simulink model "Timer"  (R2019b)
settings: Solver=VariableStepAuto  StartTime=0.0  StopTime=10.0  RelTol=1e-3
libraries: powerlib_meascontrol x1
settings Model: Creator=YJR  LastModifiedBy=YJR

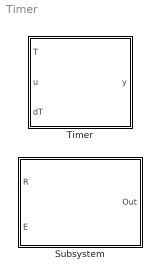
== system Timer ==
  Subsystem : Subsystem  mask(CounterEnabled){}
      mask help: Count the number of square waves.
      mask Display: disp('CounterEnabled')
  Timer : Subsystem  mask(Time Count){}
      mask help: The timer starts when it is triggered, and it is output after a set time. You can set the duration and time step.
      mask Display: disp('Timer')

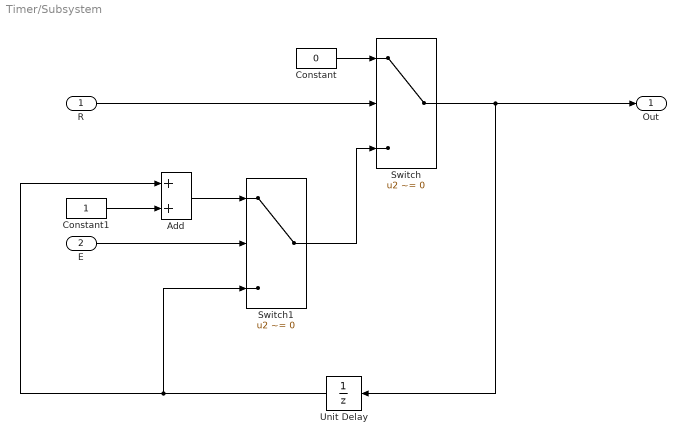
== system Timer/Subsystem ==
  R : Inport
  E : Inport  Port=2
  Add : Sum
  Constant : Constant  Value=0
  Constant1 : Constant
  Switch : Switch  Criteria=u2 ~= 0
  Switch1 : Switch  Criteria=u2 ~= 0
  Unit Delay : UnitDelay  SampleTime=-1  HasFrameUpgradeWarning=on
  Out : Outport
  wires:
  Constant/1 -> Switch/1
  Switch1/1 -> Switch/3
  Switch/1 -> Out/1, Unit Delay/1
  Add/1 -> Switch1/1
  R/1 -> Switch/2
  E/1 -> Switch1/2
  Unit Delay/1 -> Switch1/3, Add/1
  Constant1/1 -> Add/2

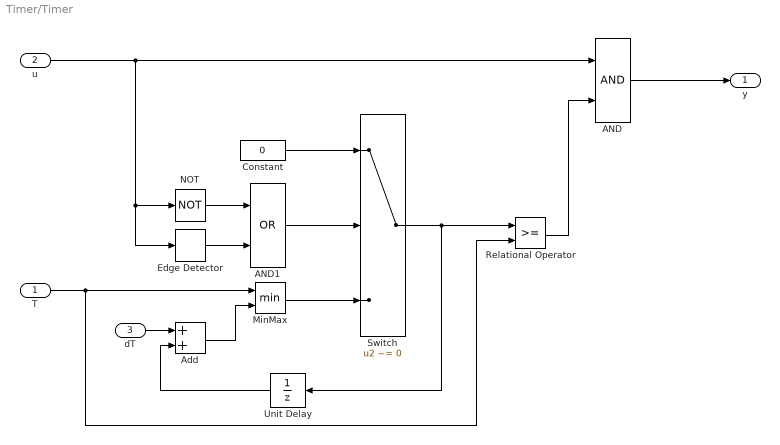
== system Timer/Timer ==
  T : Inport
  u : Inport  Port=2
  dT : Inport  Port=3
  AND : Logic  AllPortsSameDT=off  OutDataTypeStr=boolean
  AND1 : Logic  Operator=OR  AllPortsSameDT=off  OutDataTypeStr=boolean
  Add : Sum
  Constant : Constant  Value=0
  Edge Detector : powerlib_meascontrol/Logic/Edge Detector  model=Rising  ic=0  Ts=-1
      settings: SourceProductName=Simscape Electrical  SourceProductBaseCode=PS
  MinMax : MinMax  Inputs=2
  NOT : Logic  Operator=NOT  AllPortsSameDT=off  OutDataTypeStr=boolean
  Relational Operator : RelationalOperator  OutDataTypeStr=boolean  RndMeth=Simplest
  Switch : Switch  Criteria=u2 ~= 0
  Unit Delay : UnitDelay  SampleTime=-1  HasFrameUpgradeWarning=on
  y : Outport
  wires:
  Edge Detector/1 -> AND1/2
  u/1 -> Edge Detector/1, NOT/1, AND/1
  AND/1 -> y/1
  Unit Delay/1 -> Add/2
  Add/1 -> MinMax/2
  dT/1 -> Add/1
  Switch/1 -> Relational Operator/1, Unit Delay/1
  NOT/1 -> AND1/1
  T/1 -> MinMax/1, Relational Operator/2
  Constant/1 -> Switch/1
  AND1/1 -> Switch/2
  MinMax/1 -> Switch/3
  Relational Operator/1 -> AND/2
